simulink model "LaneCenterCoordChange"  (R2024a)
settings: configuration reference "csMultiInstance" (kept outside this file)
undefined symbols (not defined in the file or in its folder): Ts
Description:
  | Software unit for lane center coordinate change
settings Model: DataDictionary=DD_LaneCenterCoordChange.sldd  EnableAccessToBaseWorkspace=off  Creator=The MathWorks, Inc.  LastModifiedBy=The MathWorks, Inc.
settings ConfigSetRef: SourceName=csMultiInstance

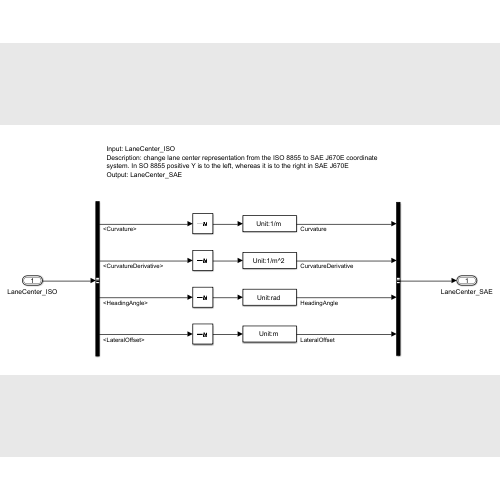
[thumbnail: Simulink's stored preview of the top-level diagram]
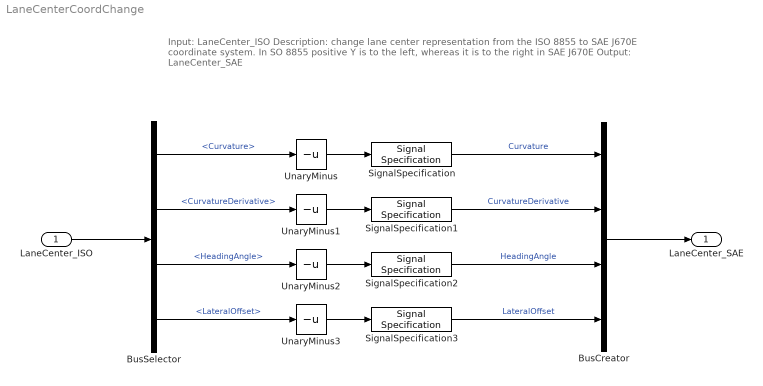
== system LaneCenterCoordChange ==
  note: Input: LaneCenter_ISO
      | Description: change lane center representation from the ISO 8855 to SAE J670E coordinate system. In SO 8855 positive Y is to the left, whereas it is to the right in SAE J670E
      | Output: LaneCenter_SAE
  LaneCenter_ISO : Inport  OutDataTypeStr=Bus: BusLaneCenter  PortDimensions=1  SampleTime=Ts
  BusCreator : BusCreator  Inputs=4  OutDataTypeStr=Bus: BusLaneCenter
  BusSelector : BusSelector  OutputSignals=Curvature,CurvatureDerivative,HeadingAngle,LateralOffset
  SignalSpecification : SignalSpecification  Unit=1/m
  SignalSpecification1 : SignalSpecification  Unit=1/m^2
  SignalSpecification2 : SignalSpecification  Unit=rad
  SignalSpecification3 : SignalSpecification  Unit=m
  UnaryMinus{,1..3} (4 alike) : UnaryMinus
  LaneCenter_SAE : Outport  OutDataTypeStr=Bus: BusLaneCenter  PortDimensions=1  SampleTime=Ts  VectorParamsAs1DForOutWhenUnconnected=off
  wires:
  SignalSpecification3/1 -> BusCreator/4  "LateralOffset"
  LaneCenter_ISO/1 -> BusSelector/1
  BusSelector/1 -> UnaryMinus/1  "<Curvature>"
  BusSelector/2 -> UnaryMinus1/1  "<CurvatureDerivative>"
  UnaryMinus2/1 -> SignalSpecification2/1
  UnaryMinus1/1 -> SignalSpecification1/1
  SignalSpecification/1 -> BusCreator/1  "Curvature"
  BusSelector/3 -> UnaryMinus2/1  "<HeadingAngle>"
  UnaryMinus/1 -> SignalSpecification/1
  UnaryMinus3/1 -> SignalSpecification3/1
  BusSelector/4 -> UnaryMinus3/1  "<LateralOffset>"
  SignalSpecification1/1 -> BusCreator/2  "CurvatureDerivative"
  SignalSpecification2/1 -> BusCreator/3  "HeadingAngle"
  BusCreator/1 -> LaneCenter_SAE/1
